simulink model "inv_dyn_joint_space"  (R2023a)
settings: Solver=VariableStepAuto  StartTime=0.0  StopTime=1  RelTol=1e-3
undefined symbols (not defined in the file): dqi, hat_flag, KD, KP, qi, robot
settings Model: Creator=franc  LastModifiedBy=franc

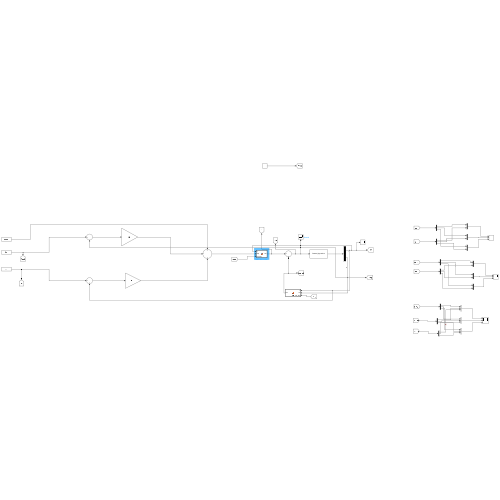
[thumbnail: Simulink's stored preview of the top-level diagram]
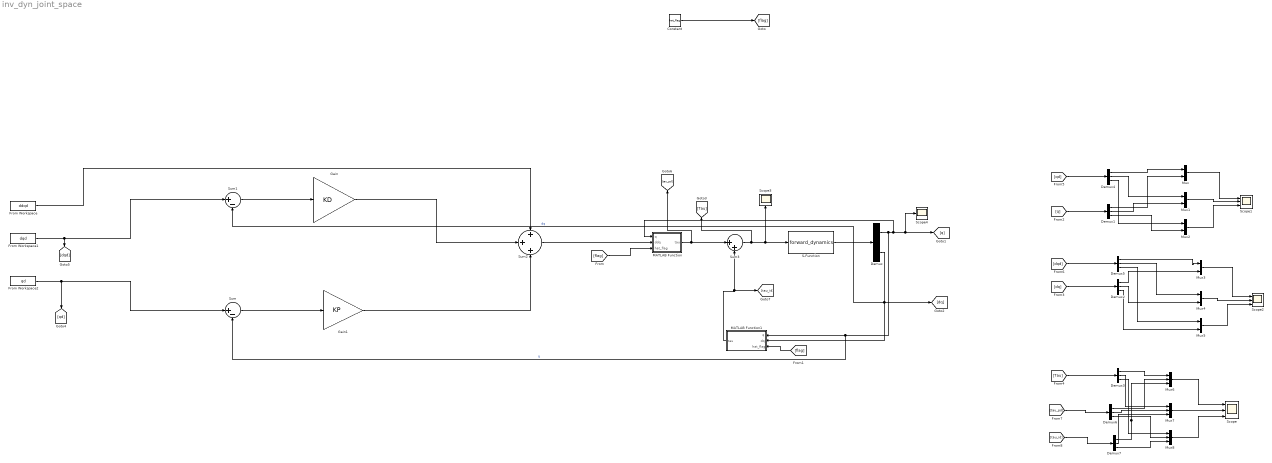
== system inv_dyn_joint_space ==
  Constant : Constant  Value=hat_flag
  Demux : Demux  Outputs=2
  Demux{1..7} (7 alike) : Demux  Outputs=3
  From Workspace : FromWorkspace  VariableName=ddqd
  From Workspace1 : FromWorkspace  VariableName=dqd
  From Workspace2 : FromWorkspace  VariableName=qd
  Gain : Gain  Gain=KD
  Gain1 : Gain  Gain=KP
  MATLAB Function : MATLAB Function  TreatAsAtomicUnit=on
  MATLAB Function1 : MATLAB Function  TreatAsAtomicUnit=on
  Mux{,1..5} (6 alike) : Mux  Inputs=2
  Mux6 : Mux  Inputs=3
  Mux7 : Mux  Inputs=3
  Mux8 : Mux  Inputs=3
  S-Function : S-Function  FunctionName=forward_dynamics  Parameters=robot,qi,dqi  SFunctionDeploymentMode=off  EnableBusSupport=off
  Scope : Scope  NumInputPorts=3
  Scope1 : Scope  NumInputPorts=3
  Scope2 : Scope  NumInputPorts=3
  Scope3 : Scope
  Scope4 : Scope
  Sum : Sum  Inputs=|+-
  Sum1 : Sum  Inputs=|+-
  Sum2 : Sum  Inputs=+++
  Sum3 : Sum  Inputs=|++
  wires:
  From Workspace1/1 -> [dqd], Sum1/1
  From Workspace2/1 -> [qd], Sum/1
  Gain/1 -> Sum2/2
  Gain1/1 -> Sum2/3
  From Workspace/1 -> Sum2/1
  Sum1/1 -> Gain/1
  Sum/1 -> Gain1/1
  Sum2/1 -> MATLAB Function/2(ddq)
  Sum3/1 -> S-Function/1, Scope3/1, [Tau]
  S-Function/1 -> Demux/1
  Demux/1 -> MATLAB Function/1(q), Scope4/1, [q], Sum/2, MATLAB Function1/1(q)  "q"
  Demux/2 -> Sum1/2, [dq], MATLAB Function1/2(dq)  "dq"
  Constant/1 -> [flag]
  [flag] -> MATLAB Function/3(hat_flag)
  [flag] -> MATLAB Function1/3(hat_flag)
  [q] -> Demux1/1
  [dq] -> Demux2/1
  [Tau] -> Demux3/1
  [qd] -> Demux4/1
  [dqd] -> Demux5/1
  Demux4/1 -> Mux/1
  Demux1/1 -> Mux/2
  Demux4/2 -> Mux1/1
  Demux4/3 -> Mux2/1
  Demux1/2 -> Mux1/2
  Demux1/3 -> Mux2/2
  Mux/1 -> Scope1/1
  Mux1/1 -> Scope1/2
  Mux2/1 -> Scope1/3
  Mux4/1 -> Scope2/2
  Mux3/1 -> Scope2/1
  Mux5/1 -> Scope2/3
  Demux5/1 -> Mux3/1
  Demux5/2 -> Mux4/1
  Demux5/3 -> Mux5/1
  Demux2/1 -> Mux3/2
  Demux2/2 -> Mux4/2
  Demux2/3 -> Mux5/2
  MATLAB Function/1(tau) -> Sum3/1, [tau_pd]
  MATLAB Function1/1(tau) -> [tau_id], Sum3/2
  [tau_id] -> Demux7/1
  [tau_pd] -> Demux6/1
  Demux3/1 -> Mux6/1
  Demux6/1 -> Mux6/2
  Demux7/1 -> Mux6/3
  Demux3/2 -> Mux7/1
  Demux6/2 -> Mux7/2
  Demux7/2 -> Mux7/3
  Demux3/3 -> Mux8/1
  Demux6/3 -> Mux8/2
  Demux7/3 -> Mux8/3
  Mux6/1 -> Scope/1
  Mux7/1 -> Scope/2
  Mux8/1 -> Scope/3

== matlab function inv_dyn_joint_space/MATLAB Function ==
  data: q input; tau output; ddq input; hat_flag input
function tau = B(q,ddq,hat_flag)

if hat_flag == 0
    B = get_B_as_7(q(1),q(3));
else
    B = get_B_hat_as_7(q(1),q(3));
end
tau = B * ddq;

== matlab function inv_dyn_joint_space/MATLAB Function1 ==
  data: q input; tau output; dq input; hat_flag input
function tau = N(q, dq, hat_flag)
tau = zeros(3,1);
if hat_flag == 0
    tau = get_n_as_7(q(1),q(3),dq(1),dq(3));
else
    tau = get_n_hat_as_7(q(1),q(3),dq(1),dq(3));
end
